simulink subsystem "iLBCReceive"  (R2024b)
settings: Solver=VariableStepAuto  StartTime=0.0  StopTime=10.0  RelTol=1e-3
undefined symbols (not defined in the file or in its folder): ilbc, ilbcMode, Newton, Raphson
libraries: simulink x15, matrix_library x6, dspilbclib x3, dspstat3 x3, dspquant2 x3, dspsigops x2, dspsnks4 x1, simulink_need_slupdate x1, dspobslib x1
settings Model: Creator=fredr  LastModifiedBy=fredr

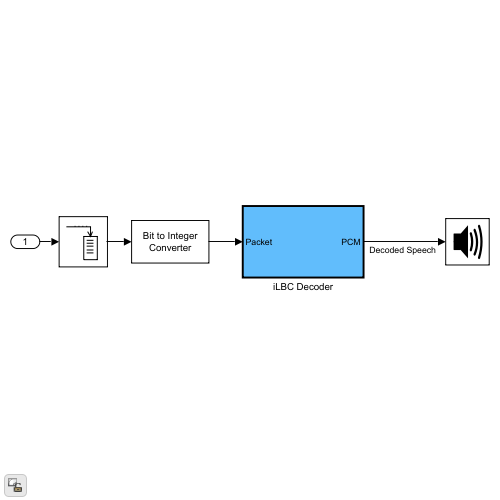
[thumbnail: Simulink's stored preview of the top-level diagram]
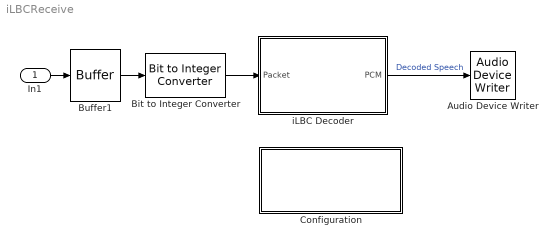
== system iLBCReceive ==
  In1 : Inport
  Audio Device Writer : dspsnks4/Audio Device Writer  Driver=DirectSound  Device=Default  InheritSampleRate=off  SampleRate=8000  BitDepth=16-bit integer  BufferSize=4096  NumBuffers=10  DefaultOutputChannelMapping=on  OutputChannelMapping=1:2  OutputNumUnderrunSamples=off  DriverIdx=1  DeviceWarnFlag=''
  Bit to Integer Converter : simulink/Logic and Bit Operations/Bit to Integer Converter  nbits=8  bitOrder=MSB first  signedOutputValues=Unsigned  outDtype=Inherit via internal rule  outDtypeSigned=Inherit via internal rule
  Buffer1 : Buffer  N=400  OutputFrames=off
  Configuration : Subsystem  mask(iLBC Configuration){ilbcDialogMode=13.33 kbit/sec mode, ilbcDialogDatatype=double}
      mask prompts: ilbcDialogMode "iLBC mode:"; ilbcDialogDatatype "Internal data type:"
      mask help:
      | The iLBC standard is defined for two data rates: 13.33 kbit/sec and 15.20 kbit/sec.  Running under 13.33 kbit/sec, the encoder creates and outputs a compressed speech packet every 30ms.  With the 15.20 kbit/sec data rate, the encoder will output a packet every 20ms.  For the 13.33 kbit/sec mode, the packet size is a uint8 column vector of length 50, where each element represents one byte.  For the 15.20 kbit/sec mode, the packet is of length 38 bytes.
      |
      | The "Internal Data Type" option controls the precision for all internal floating point calculations in the iLBC Encoder and Decoder. The possible options are double and single precision.
      mask init:
      | if ilbcDialogMode == 1
      |     ilbcModeStr = '13.33';
      | elseif ilbcDialogMode == 2
      |     ilbcModeStr = '15.20';
      | end
      | 
      | if ilbcDialogDatatype == 1
      |     ilbcDatatype = 'double';
      | elseif ilbcDialogDatatype == 2
      |     ilbcDatatype = 'single';
      | end
      mask TypeOptions ilbcDialogMode: 13.33 kbit/sec mode | 15.20 kbit/sec mode
      mask TypeOptions ilbcDialogDatatype: double | single
      mask Display:
      | disp([ilbcModeStr ' kb/sec mode\n' ...
      |     'Internal data type: ' ilbcDatatype '\n' ...
      |     '[Double-click to change]']);
  iLBC Decoder : Subsystem  TreatAsAtomicUnit=on
  wires:
  Buffer1/1 -> Bit to Integer Converter/1
  iLBC Decoder/1(PCM) -> Audio Device Writer/1  "Decoded Speech"
  Bit to Integer Converter/1 -> iLBC Decoder/1(Packet)
  In1/1 -> Buffer1/1

== system iLBCReceive/Configuration ==

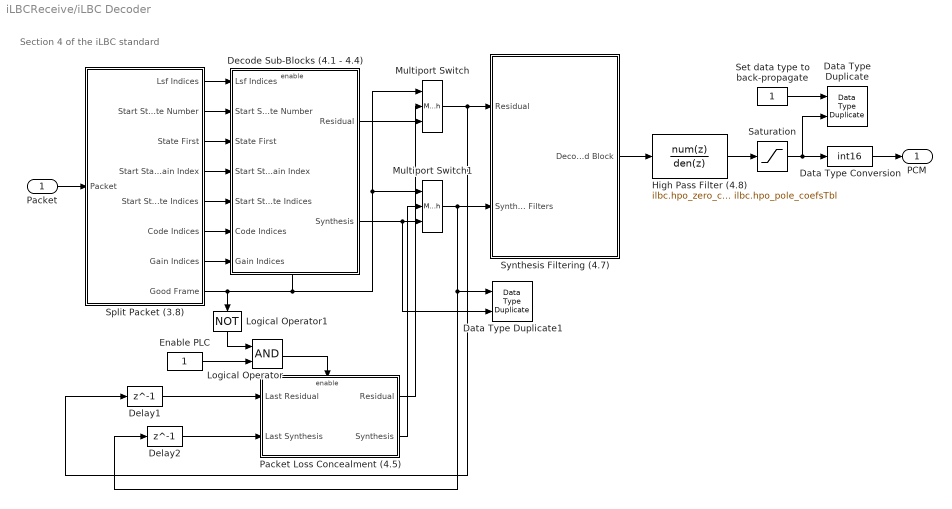
== system iLBCReceive/iLBC Decoder ==
  note: Section 4 of the iLBC standard
  Packet : Inport
  Data Type Duplicate : DataTypeDuplicate
  Data Type Duplicate1 : DataTypeDuplicate
  Data Type Conversion : DataTypeConversion  OutDataTypeStr=int16  RndMeth=Floor
  Decode Sub-Blocks (4.1 - 4.4) : Subsystem
  Delay1 : Delay  DelayLength=1  InitialCondition=0
  Delay2 : Delay  DelayLength=1  InitialCondition=0
  Enable PLC : Constant  OutDataTypeStr=boolean
  High Pass Filter (4.8) : DiscreteFilter  Numerator=ilbc.hpo_zero_coefsTbl  Denominator=ilbc.hpo_pole_coefsTbl  InputProcessing=Columns as channels (frame based)  FilterStructure=Direct form II transposed  a0EqualsOne=on  NumAccumDataTypeStr=Inherit: Same as product output  DenAccumDataTypeStr=Inherit: Same as product output
  Logical Operator : Logic  AllPortsSameDT=off  OutDataTypeStr=boolean
  Logical Operator1 : Logic  Operator=NOT  AllPortsSameDT=off  OutDataTypeStr=boolean
  Multiport Switch : MultiPortSwitch  DataPortOrder=Zero-based contiguous  Inputs=2  zeroidx=on  SaturateOnIntegerOverflow=off  InputSameDT=off
  Multiport Switch1 : MultiPortSwitch  DataPortOrder=Zero-based contiguous  Inputs=2  zeroidx=on  SaturateOnIntegerOverflow=off  InputSameDT=off
  Packet Loss Concealment (4.5) : Subsystem
  Saturation : Saturate  UpperLimit=32767  LowerLimit=-32768
  Set data type to back-propagate : Constant  OutDataTypeStr=ilbcDatatype
  Split Packet (3.8) : Subsystem  TreatAsAtomicUnit=on
  Synthesis Filtering (4.7) : Subsystem  TreatAsAtomicUnit=on
  PCM : Outport  VectorParamsAs1DForOutWhenUnconnected=off
  wires:
  Delay2/1 -> Packet Loss Concealment (4.5)/2(Last Synthesis)
  Multiport Switch1/1 -> Synthesis Filtering (4.7)/2(Synthesis Filters), Data Type Duplicate1/1, Delay2/1
  Delay1/1 -> Packet Loss Concealment (4.5)/1(Last Residual)
  Multiport Switch/1 -> Synthesis Filtering (4.7)/1(Residual), Delay1/1
  High Pass Filter (4.8)/1 -> Saturation/1
  Packet/1 -> Split Packet (3.8)/1(Packet)
  Data Type Conversion/1 -> PCM/1
  Saturation/1 -> Data Type Conversion/1, Data Type Duplicate/2
  Synthesis Filtering (4.7)/1(Decoded Block) -> High Pass Filter (4.8)/1
  Split Packet (3.8)/2(Start State Number) -> Decode Sub-Blocks (4.1 - 4.4)/2(Start State Number)
  Split Packet (3.8)/3(State First) -> Decode Sub-Blocks (4.1 - 4.4)/3(State First)
  Split Packet (3.8)/4(Start State Gain Index) -> Decode Sub-Blocks (4.1 - 4.4)/4(Start State Gain Index)
  Split Packet (3.8)/5(Start State Indices) -> Decode Sub-Blocks (4.1 - 4.4)/5(Start State Indices)
  Split Packet (3.8)/6(Code Indices) -> Decode Sub-Blocks (4.1 - 4.4)/6(Code Indices)
  Split Packet (3.8)/7(Gain Indices) -> Decode Sub-Blocks (4.1 - 4.4)/7(Gain Indices)
  Split Packet (3.8)/1(Lsf Indices) -> Decode Sub-Blocks (4.1 - 4.4)/1(Lsf Indices)
  Split Packet (3.8)/8(Good Frame) -> Logical Operator1/1, Multiport Switch/1, Multiport Switch1/1, Decode Sub-Blocks (4.1 - 4.4)/Enable
  Decode Sub-Blocks (4.1 - 4.4)/1(Residual) -> Multiport Switch/3
  Decode Sub-Blocks (4.1 - 4.4)/2(Synthesis) -> Multiport Switch1/3, Data Type Duplicate1/2
  Packet Loss Concealment (4.5)/1(Residual) -> Multiport Switch/2
  Packet Loss Concealment (4.5)/2(Synthesis) -> Multiport Switch1/2
  Logical Operator/1 -> Packet Loss Concealment (4.5)/Enable
  Logical Operator1/1 -> Logical Operator/1
  Set data type to back-propagate/1 -> Data Type Duplicate/1
  Enable PLC/1 -> Logical Operator/2

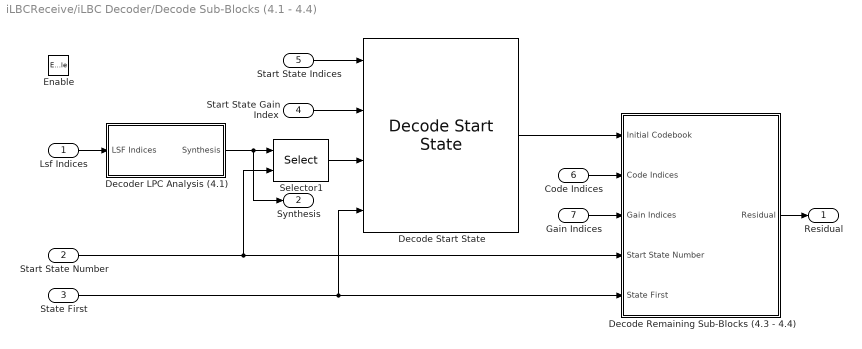
== system iLBCReceive/iLBC Decoder/Decode Sub-Blocks (4.1 - 4.4) ==
  Lsf Indices : Inport
  Start State Number : Inport  Port=2
  State First : Inport  Port=3
  Start State Gain Index : Inport  Port=4
  Start State Indices : Inport  Port=5
  Code Indices : Inport  Port=6
  Gain Indices : Inport  Port=7
  Enable : EnablePort
  Decode Remaining Sub-Blocks (4.3 - 4.4) : Subsystem  TreatAsAtomicUnit=on
  Decode Start State : dspilbclib/Decode Start State  SystemSampleTime=-1  VariantActivationTime=update diagram  AllowFlexibleInterface=on  Latency=0  AutoFrameSizeCalculation=off
  Decoder LPC Analysis (4.1) : Subsystem  TreatAsAtomicUnit=on
  Selector1 : Selector  NumberOfDimensions=2  InputPortWidth=3  IndexOptions=Select all,Index vector (port)  Indices=-1,-1  OutputSizes=1
  Residual : Outport  VectorParamsAs1DForOutWhenUnconnected=off
  Synthesis : Outport  Port=2  VectorParamsAs1DForOutWhenUnconnected=off
  wires:
  Decode Remaining Sub-Blocks (4.3 - 4.4)/1(Residual) -> Residual/1
  Gain Indices/1 -> Decode Remaining Sub-Blocks (4.3 - 4.4)/3(Gain Indices)
  Code Indices/1 -> Decode Remaining Sub-Blocks (4.3 - 4.4)/2(Code Indices)
  Start State Gain Index/1 -> Decode Start State/2
  Start State Indices/1 -> Decode Start State/1
  Decoder LPC Analysis (4.1)/1(Synthesis) -> Selector1/1, Synthesis/1
  Lsf Indices/1 -> Decoder LPC Analysis (4.1)/1(LSF Indices)
  State First/1 -> Decode Remaining Sub-Blocks (4.3 - 4.4)/5(State First), Decode Start State/4
  Selector1/1 -> Decode Start State/3
  Start State Number/1 -> Decode Remaining Sub-Blocks (4.3 - 4.4)/4(Start State Number), Selector1/2
  Decode Start State/1 -> Decode Remaining Sub-Blocks (4.3 - 4.4)/1(Initial Codebook)

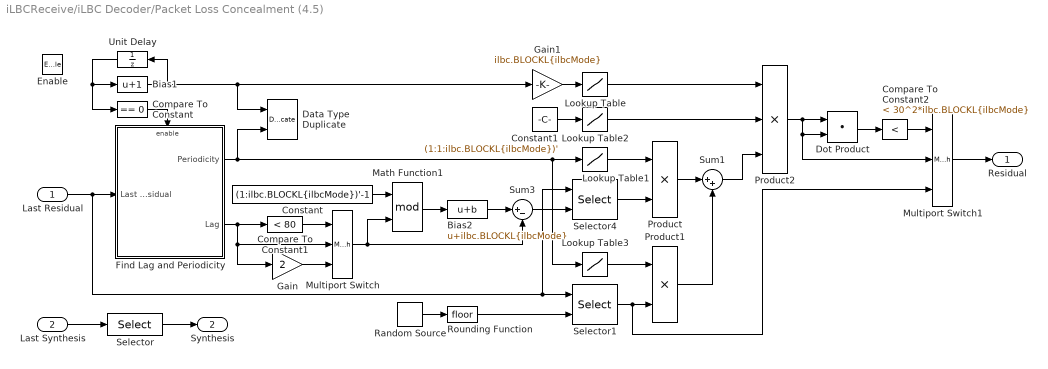
== system iLBCReceive/iLBC Decoder/Packet Loss Concealment (4.5) ==
  Last Residual : Inport
  Last Synthesis : Inport  Port=2
  Enable : EnablePort  StatesWhenEnabling=reset
  Bias1 : Bias  Bias=1  SaturateOnIntegerOverflow=off
  Bias2 : Bias  Bias=ilbc.BLOCKL{ilbcMode}  SaturateOnIntegerOverflow=off
  Compare To Constant : simulink/Logic and Bit Operations/Compare To Constant  relop===  const=0  OutDataTypeStr=boolean  ZeroCross=off
  Compare To Constant1 : simulink/Logic and Bit Operations/Compare To Constant  relop=<  const=80  OutDataTypeStr=uint8  ZeroCross=off
  Compare To Constant2 : simulink/Logic and Bit Operations/Compare To Constant  relop=<  const=30^2*ilbc.BLOCKL{ilbcMode}  OutDataTypeStr=boolean  ZeroCross=off
  Constant : Constant  Value=(1:ilbc.BLOCKL{ilbcMode})'-1  VectorParams1D=off  OutDataTypeStr=Inherit: Inherit via back propagation
  Constant1 : Constant  Value=(1:1:ilbc.BLOCKL{ilbcMode})'  VectorParams1D=off  OutDataTypeStr=Inherit: Inherit via back propagation
  Data Type Duplicate : DataTypeDuplicate
  Dot Product : DotProduct  OutDataTypeStr=Inherit: Inherit via internal rule
  Find Lag and Periodicity : Subsystem  TreatAsAtomicUnit=on
  Gain : Gain  Gain=2  OutDataTypeStr=Inherit: Same as input
  Gain1 : Gain  Gain=ilbc.BLOCKL{ilbcMode}  OutDataTypeStr=Inherit: Inherit via back propagation  ParamDataTypeStr=Inherit: Same as input
  Lookup Table : Lookup_n-D  NumberOfTableDimensions=1  BreakpointsForDimension1=[0 320 640 960 1280]  Table=[1.0 0.9 0.7 0.5 0.0]  InterpMethod=Flat
  Lookup Table1 : Lookup_n-D  NumberOfTableDimensions=1  BreakpointsForDimension1=[0.3 0.6]  Table=[0 1]  ExtrapMethod=Clip
  Lookup Table2 : Lookup_n-D  NumberOfTableDimensions=1  BreakpointsForDimension1=[80 160 240]  Table=[1.00 0.95 0.90]  ExtrapMethod=Clip
  Lookup Table3 : Lookup_n-D  NumberOfTableDimensions=1  BreakpointsForDimension1=[0.3 0.6]  Table=[1 0]  ExtrapMethod=Clip
  Math Function1 : Math  Operator=mod  SignedPower=on
  Multiport Switch : MultiPortSwitch  DataPortOrder=Zero-based contiguous  Inputs=2  zeroidx=on  SaturateOnIntegerOverflow=off  InputSameDT=off
  Multiport Switch1 : MultiPortSwitch  DataPortOrder=Zero-based contiguous  Inputs=2  zeroidx=on  SaturateOnIntegerOverflow=off  InputSameDT=off
  Product : Product  RndMeth=Zero
  Product1 : Product  RndMeth=Zero
  Product2 : Product  Inputs=3  RndMeth=Zero  OutDataTypeStr=Inherit: Same as first input
  Random Source : dspobslib/Random Source  SrcType=Uniform  NormMethod=Ziggurat  CltLength=12  MinVal=ilbc.BLOCKL{ilbcMode}-70  MaxVal=ilbc.BLOCKL{ilbcMode}-0.001  MeanVal=0  VarVal=1  RepMode=Not repeatable  rawSeed=1  IsInherit=off  SampMode=Discrete  SampTime=-1  SampFrame=ilbc.BLOCKL{ilbcMode}  DataType=Single  OutComplex=Real  OutputFrames=off
  Rounding Function : Rounding
  Selector : Selector  NumberOfDimensions=2  InputPortWidth=3  IndexOptions=Select all,Index vector (dialog)  Indices=[1 3],repmat(ilbc.NSUB{ilbcMode},1,ilbc.NSUB{ilbcMode})  OutputSizes=1,1
  Selector1 : Selector  NumberOfDimensions=2  IndexMode=Zero-based  InputPortWidth=3  IndexOptions=Index vector (port),Select all  Indices=[1 3],1  OutputSizes=1,1
  Selector4 : Selector  NumberOfDimensions=2  IndexMode=Zero-based  InputPortWidth=3  IndexOptions=Index vector (port),Select all  Indices=[1 3],1  OutputSizes=1,1
  Sum1 : Sum  Inputs=|++
  Sum3 : Sum  Inputs=|+-
  Unit Delay : UnitDelay  SampleTime=-1  HasFrameUpgradeWarning=on
  Residual : Outport  VectorParamsAs1DForOutWhenUnconnected=off
  Synthesis : Outport  Port=2  VectorParamsAs1DForOutWhenUnconnected=off
  wires:
  Last Synthesis/1 -> Selector/1
  Selector/1 -> Synthesis/1
  Find Lag and Periodicity/2(Lag) -> Compare To Constant1/1, Multiport Switch/2, Gain/1
  Find Lag and Periodicity/1(Periodicity) -> Lookup Table1/1, Lookup Table3/1, Data Type Duplicate/2
  Compare To Constant1/1 -> Multiport Switch/1
  Gain1/1 -> Lookup Table/1
  Constant1/1 -> Lookup Table2/1
  Sum1/1 -> Product2/3
  Dot Product/1 -> Compare To Constant2/1
  Compare To Constant2/1 -> Multiport Switch1/1
  Multiport Switch1/1 -> Residual/1
  Lookup Table/1 -> Product2/1
  Lookup Table2/1 -> Product2/2
  Last Residual/1 -> Find Lag and Periodicity/1(Last Residual), Selector4/1, Selector1/1
  Product2/1 -> Dot Product/1, Dot Product/2, Multiport Switch1/2
  Constant/1 -> Math Function1/1
  Math Function1/1 -> Bias2/1
  Bias2/1 -> Sum3/1
  Sum3/1 -> Selector4/2
  Multiport Switch/1 -> Math Function1/2, Sum3/2
  Lookup Table1/1 -> Product/1
  Selector4/1 -> Product/2
  Lookup Table3/1 -> Product1/1
  Selector1/1 -> Product1/2, Multiport Switch1/3
  Product/1 -> Sum1/1
  Product1/1 -> Sum1/2
  Gain/1 -> Multiport Switch/3
  Random Source/1 -> Rounding Function/1
  Compare To Constant/1 -> Find Lag and Periodicity/Enable
  Unit Delay/1 -> Bias1/1, Compare To Constant/1
  Rounding Function/1 -> Selector1/2
  Bias1/1 -> Unit Delay/1, Gain1/1, Data Type Duplicate/1

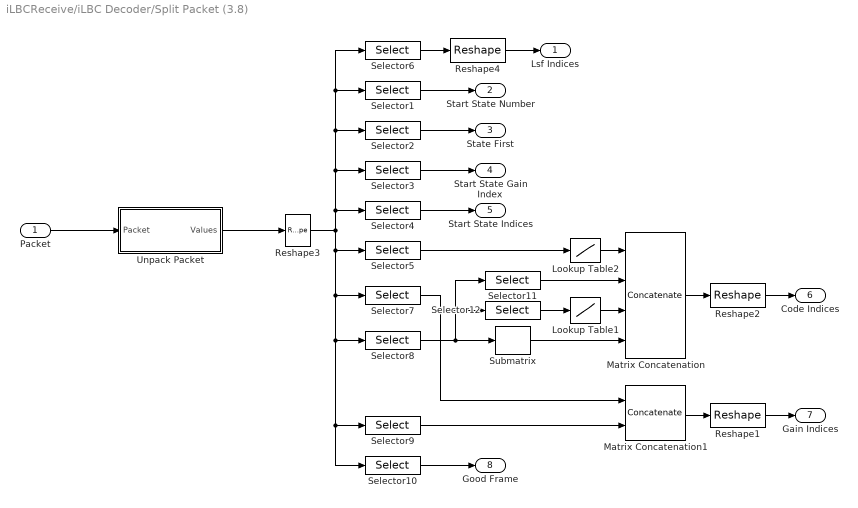
== system iLBCReceive/iLBC Decoder/Split Packet (3.8) ==
  Packet : Inport
  Lookup Table1 : Lookup_n-D  NumberOfTableDimensions=1  BreakpointsForDimension1=[0:255]  Table=[0:43 108:171 236:255 zeros(1,128)]  ExtrapMethod=Clip
  Lookup Table2 : Lookup_n-D  NumberOfTableDimensions=1  BreakpointsForDimension1=[0:255]  Table=[0:57 zeros(1,6) 128:185 zeros(1,134)]  ExtrapMethod=Clip
  Matrix Concatenation : Concatenate  NumInputs=4  Mode=Multidimensional array
  Matrix Concatenation1 : Concatenate  Mode=Multidimensional array
  Reshape1 : Reshape  OutputDimensionality=Customize  OutputDimensions=[3 (ilbc.NSUB{ilbcMode}-1)]
  Reshape2 : Reshape  OutputDimensionality=Customize  OutputDimensions=[3 (ilbc.NSUB{ilbcMode}-1)]
  Reshape3 : Reshape  OutputDimensionality=Column vector (2-D)
  Reshape4 : Reshape  OutputDimensionality=Customize  OutputDimensions=[3 (3-ilbcMode)]
  Selector1 : Selector  NumberOfDimensions=2  InputPortWidth=3  IndexOptions=Index vector (dialog),Select all  Indices=ilbc.packet_idxTbl{ilbcMode}{2},-1  OutputSizes=1
  Selector10 : Selector  NumberOfDimensions=2  InputPortWidth=3  IndexOptions=Index vector (dialog),Select all  Indices=ilbc.packet_idxTbl{ilbcMode}{10},-1  OutputSizes=1
  Selector11 : Selector  NumberOfDimensions=2  InputPortWidth=3  IndexOptions=Index vector (dialog),Select all  Indices=1,-1  OutputSizes=1
  Selector12 : Selector  NumberOfDimensions=2  InputPortWidth=3  IndexOptions=Index vector (dialog),Select all  Indices=2:3,-1  OutputSizes=1
  Selector2 : Selector  NumberOfDimensions=2  InputPortWidth=3  IndexOptions=Index vector (dialog),Select all  Indices=ilbc.packet_idxTbl{ilbcMode}{3},-1  OutputSizes=1
  Selector3 : Selector  NumberOfDimensions=2  InputPortWidth=3  IndexOptions=Index vector (dialog),Select all  Indices=ilbc.packet_idxTbl{ilbcMode}{4},-1  OutputSizes=1
  Selector4 : Selector  NumberOfDimensions=2  InputPortWidth=3  IndexOptions=Index vector (dialog),Select all  Indices=ilbc.packet_idxTbl{ilbcMode}{5},-1  OutputSizes=1
  Selector5 : Selector  NumberOfDimensions=2  InputPortWidth=3  IndexOptions=Index vector (dialog),Select all  Indices=ilbc.packet_idxTbl{ilbcMode}{6},-1  OutputSizes=1
  Selector6 : Selector  NumberOfDimensions=2  InputPortWidth=3  IndexOptions=Index vector (dialog),Select all  Indices=ilbc.packet_idxTbl{ilbcMode}{1},-1  OutputSizes=1
  Selector7 : Selector  NumberOfDimensions=2  InputPortWidth=3  IndexOptions=Index vector (dialog),Select all  Indices=ilbc.packet_idxTbl{ilbcMode}{7},-1  OutputSizes=1
  Selector8 : Selector  NumberOfDimensions=2  InputPortWidth=3  IndexOptions=Index vector (dialog),Select all  Indices=ilbc.packet_idxTbl{ilbcMode}{8},-1  OutputSizes=1
  Selector9 : Selector  NumberOfDimensions=2  InputPortWidth=3  IndexOptions=Index vector (dialog),Select all  Indices=ilbc.packet_idxTbl{ilbcMode}{9},-1  OutputSizes=1
  Submatrix : matrix_library/Submatrix  RowSpan=Range of rows  RowStartMode=Index  RowStartIndex=4  RowEndMode=Last  RowEndIndex=1  ColSpan=All columns  ColStartMode=First  ColStartIndex=1  ColEndMode=Last  ColEndIndex=1
  Unpack Packet : Subsystem  TreatAsAtomicUnit=on
  Lsf Indices : Outport  VectorParamsAs1DForOutWhenUnconnected=off
  Start State Number : Outport  Port=2  VectorParamsAs1DForOutWhenUnconnected=off
  State First : Outport  Port=3  VectorParamsAs1DForOutWhenUnconnected=off
  Start State Gain Index : Outport  Port=4  VectorParamsAs1DForOutWhenUnconnected=off
  Start State Indices : Outport  Port=5  VectorParamsAs1DForOutWhenUnconnected=off
  Code Indices : Outport  Port=6  VectorParamsAs1DForOutWhenUnconnected=off
  Gain Indices : Outport  Port=7  VectorParamsAs1DForOutWhenUnconnected=off
  Good Frame : Outport  Port=8  VectorParamsAs1DForOutWhenUnconnected=off
  wires:
  Matrix Concatenation/1 -> Reshape2/1
  Matrix Concatenation1/1 -> Reshape1/1
  Reshape2/1 -> Code Indices/1
  Reshape1/1 -> Gain Indices/1
  Selector1/1 -> Start State Number/1
  Selector3/1 -> Start State Gain Index/1
  Selector4/1 -> Start State Indices/1
  Selector2/1 -> State First/1
  Selector9/1 -> Matrix Concatenation1/2
  Selector7/1 -> Matrix Concatenation1/1
  Selector10/1 -> Good Frame/1
  Selector6/1 -> Reshape4/1
  Reshape3/1 -> Selector8/1, Selector10/1, Selector9/1, Selector7/1, Selector5/1, Selector4/1, Selector3/1, Selector2/1, Selector6/1, Selector1/1
  Reshape4/1 -> Lsf Indices/1
  Selector5/1 -> Lookup Table2/1
  Selector8/1 -> Selector11/1, Selector12/1, Submatrix/1
  Submatrix/1 -> Matrix Concatenation/4
  Selector11/1 -> Matrix Concatenation/2
  Selector12/1 -> Lookup Table1/1
  Lookup Table2/1 -> Matrix Concatenation/1
  Lookup Table1/1 -> Matrix Concatenation/3
  Packet/1 -> Unpack Packet/1(Packet)
  Unpack Packet/1(Values) -> Reshape3/1

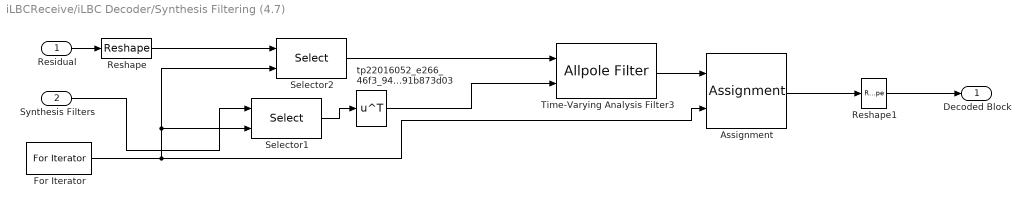
== system iLBCReceive/iLBC Decoder/Synthesis Filtering (4.7) ==
  Residual : Inport
  Synthesis Filters : Inport  Port=2
  Assignment : Assignment  NumberOfDimensions=2  OutputInitialize=Specify size for each dimension in table  IndexOptions=Assign all,Index vector (port)  Indices=-1,1  OutputSizes=40,ilbc.NSUB{ilbcMode}
  For Iterator : ForIterator  IterationLimit=ilbc.NSUB{ilbcMode}  IterationVariableDataType=int8
  Reshape : Reshape  OutputDimensionality=Customize  OutputDimensions=[40 ilbc.NSUB{ilbcMode}]
  Reshape1 : Reshape  OutputDimensionality=Column vector (2-D)  OutputDimensions=[50 4]
  Selector1 : Selector  NumberOfDimensions=2  InputPortWidth=3  IndexOptions=Select all,Index vector (port)  Indices=-1,-1  OutputSizes=1
  Selector2 : Selector  NumberOfDimensions=2  InputPortWidth=3  IndexOptions=Select all,Index vector (port)  Indices=-1,-1  OutputSizes=1
  Time-Varying Analysis Filter3 : AllpoleFilter  CoefSource=Input port  AccumDataTypeStr=Inherit: Same as product output
      settings: InputPortMap=u0,u1
  tp22016052_e266_46f3_948b_11691b873d03 : Math  Operator=transpose  SignedPower=on
  Decoded Block : Outport  VectorParamsAs1DForOutWhenUnconnected=off
  wires:
  tp22016052_e266_46f3_948b_11691b873d03/1 -> Time-Varying Analysis Filter3/2
  Selector1/1 -> tp22016052_e266_46f3_948b_11691b873d03/1
  Residual/1 -> Reshape/1
  Synthesis Filters/1 -> Selector1/1
  Selector2/1 -> Time-Varying Analysis Filter3/1
  For Iterator/1 -> Selector1/2, Selector2/2, Assignment/2
  Reshape/1 -> Selector2/1
  Time-Varying Analysis Filter3/1 -> Assignment/1
  Assignment/1 -> Reshape1/1
  Reshape1/1 -> Decoded Block/1

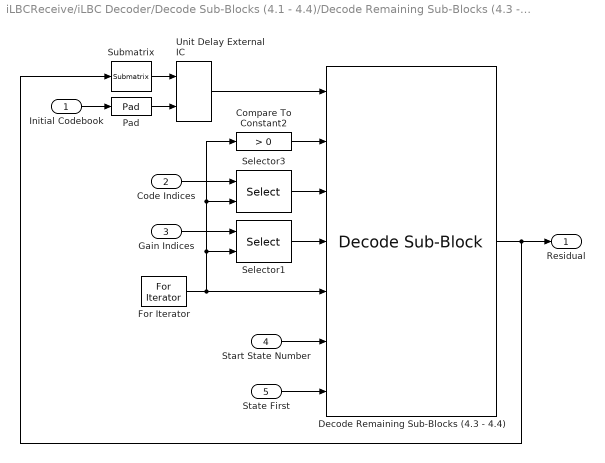
== system iLBCReceive/iLBC Decoder/Decode Sub-Blocks (4.1 - 4.4)/Decode Remaining Sub-Blocks (4.3 - 4.4) ==
  Initial Codebook : Inport
  Code Indices : Inport  Port=2
  Gain Indices : Inport  Port=3
  Start State Number : Inport  Port=4
  State First : Inport  Port=5
  Compare To Constant2 : simulink/Logic and Bit Operations/Compare To Constant  relop=>  const=0  OutDataTypeStr=uint8  ZeroCross=off
  Decode Remaining Sub-Blocks (4.3 - 4.4) : dspilbclib/Decode Sub-Block  SystemSampleTime=-1  VariantActivationTime=update diagram  AllowFlexibleInterface=on  Latency=0  AutoFrameSizeCalculation=off
  For Iterator : ForIterator  ResetStates=reset  IterationLimit=ilbc.NSUB{ilbcMode}-1  IndexMode=Zero-based
  Pad : dspsigops/Pad  padAlong=Columns  dimsToPad=1  valSrc=Specify via dialog  padVal=0  spec=Pad size  padNumOutRowsSpecMethod=User-specified  numOutRows=ilbc.BLOCKL{ilbcMode}-40  padNumOutColsSpecMethod=User-specified  numOutCols=1  isVarDimsMode=off  padBeginning=90  padEnd=0  outSizeMode=User-specified  outSize=1  padSigAt=Beginning  trunc_flag=None  roundingMode=Floor  overflowMode=off  truncOrWrapMode=Truncate  wrap_flag=None
  Selector1 : Selector  NumberOfDimensions=2  IndexMode=Zero-based  InputPortWidth=3  IndexOptions=Select all,Index vector (port)  Indices=-1,0  OutputSizes=1
  Selector3 : Selector  NumberOfDimensions=2  IndexMode=Zero-based  InputPortWidth=3  IndexOptions=Select all,Index vector (port)  Indices=-1,0  OutputSizes=1
  Submatrix : matrix_library/Submatrix  RowSpan=Range of rows  RowStartMode=Index  RowStartIndex=41  RowEndMode=Last  RowEndIndex=1  ColSpan=All columns  ColStartMode=First  ColStartIndex=1  ColEndMode=Last  ColEndIndex=1
  Unit Delay External IC : simulink_need_slupdate/Unit Delay External IC  tsamp=-1
  Residual : Outport  VectorParamsAs1DForOutWhenUnconnected=off
  wires:
  State First/1 -> Decode Remaining Sub-Blocks (4.3 - 4.4)/7
  Start State Number/1 -> Decode Remaining Sub-Blocks (4.3 - 4.4)/6
  Compare To Constant2/1 -> Decode Remaining Sub-Blocks (4.3 - 4.4)/2
  Unit Delay External IC/1 -> Decode Remaining Sub-Blocks (4.3 - 4.4)/1
  Pad/1 -> Unit Delay External IC/2
  Submatrix/1 -> Unit Delay External IC/1
  Initial Codebook/1 -> Pad/1
  Code Indices/1 -> Selector3/1
  Gain Indices/1 -> Selector1/1
  Selector1/1 -> Decode Remaining Sub-Blocks (4.3 - 4.4)/4
  Selector3/1 -> Decode Remaining Sub-Blocks (4.3 - 4.4)/3
  Decode Remaining Sub-Blocks (4.3 - 4.4)/1 -> Residual/1, Submatrix/1
  For Iterator/1 -> Decode Remaining Sub-Blocks (4.3 - 4.4)/5, Selector1/2, Compare To Constant2/1, Selector3/2

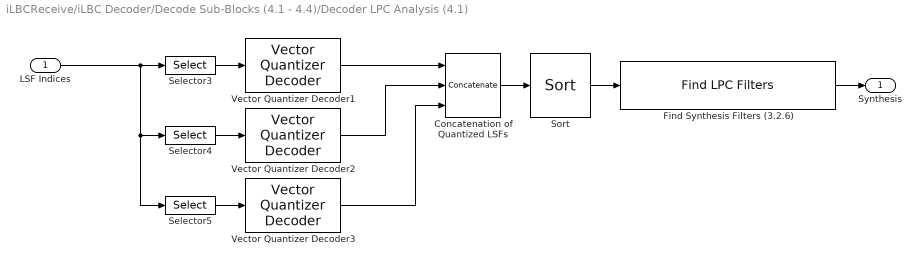
== system iLBCReceive/iLBC Decoder/Decode Sub-Blocks (4.1 - 4.4)/Decoder LPC Analysis (4.1) ==
  LSF Indices : Inport
  Concatenation of Quantized LSFs : Concatenate  NumInputs=3  Mode=Multidimensional array
  Find Synthesis Filters (3.2.6) : dspilbclib/Find LPC Filters  SystemSampleTime=-1  VariantActivationTime=update diagram  AllowFlexibleInterface=on  Latency=0  AutoFrameSizeCalculation=off
  Selector3 : Selector  NumberOfDimensions=2  InputPortWidth=3  IndexOptions=Index vector (dialog),Select all  Indices=1,-1  OutputSizes=1
  Selector4 : Selector  NumberOfDimensions=2  InputPortWidth=3  IndexOptions=Index vector (dialog),Select all  Indices=2,-1  OutputSizes=1
  Selector5 : Selector  NumberOfDimensions=2  InputPortWidth=3  IndexOptions=Index vector (dialog),Select all  Indices=3,-1  OutputSizes=1
  Sort : dspstat3/Sort  otype=Value  dir=Ascending  sortAlg=Quick sort  roundingMode=Floor  overflowMode=off
  Vector Quantizer Decoder1 : dspquant2/Vector Quantizer Decoder  invalidin=Clip  CBsource=Specify via dialog  codebook=ilbc.lsfCbTbl1  dataType=Inherit via back propagation  isSigned=on  wordLen=16  udDataType=float('single')  fracBitsMode=Best precision  numFracBits=7  OutDataTypeStr=Inherit: Inherit via back propagation  LastOutDataTypeStr=Inherit: Inherit via back propagation
  Vector Quantizer Decoder2 : dspquant2/Vector Quantizer Decoder  invalidin=Clip  CBsource=Specify via dialog  codebook=ilbc.lsfCbTbl2  dataType=Inherit via back propagation  isSigned=on  wordLen=16  udDataType=float('single')  fracBitsMode=Best precision  numFracBits=7  OutDataTypeStr=Inherit: Inherit via back propagation  LastOutDataTypeStr=Inherit: Inherit via back propagation
  Vector Quantizer Decoder3 : dspquant2/Vector Quantizer Decoder  invalidin=Clip  CBsource=Specify via dialog  codebook=ilbc.lsfCbTbl3  dataType=Inherit via back propagation  isSigned=on  wordLen=16  udDataType=float('single')  fracBitsMode=Best precision  numFracBits=7  OutDataTypeStr=Inherit: Inherit via back propagation  LastOutDataTypeStr=Inherit: Inherit via back propagation
  Synthesis : Outport  VectorParamsAs1DForOutWhenUnconnected=off
  wires:
  Selector3/1 -> Vector Quantizer Decoder1/1
  Selector4/1 -> Vector Quantizer Decoder2/1
  Selector5/1 -> Vector Quantizer Decoder3/1
  Vector Quantizer Decoder1/1 -> Concatenation of Quantized LSFs/1
  Vector Quantizer Decoder2/1 -> Concatenation of Quantized LSFs/2
  Vector Quantizer Decoder3/1 -> Concatenation of Quantized LSFs/3
  Concatenation of Quantized LSFs/1 -> Sort/1
  Sort/1 -> Find Synthesis Filters (3.2.6)/1
  Find Synthesis Filters (3.2.6)/1 -> Synthesis/1
  LSF Indices/1 -> Selector5/1, Selector4/1, Selector3/1

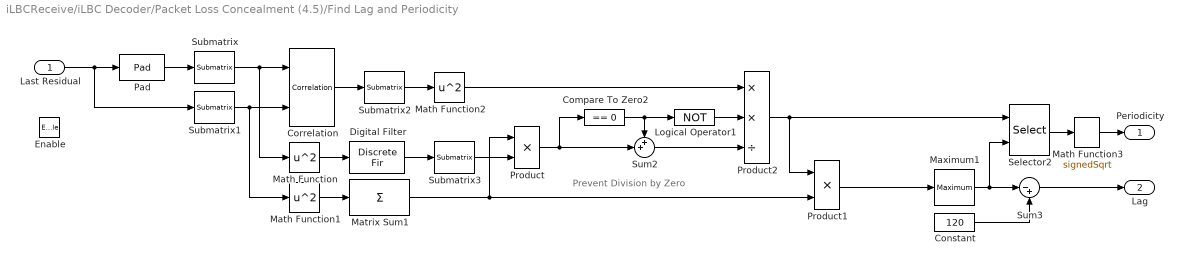
== system iLBCReceive/iLBC Decoder/Packet Loss Concealment (4.5)/Find Lag and Periodicity ==
  note: Prevent Division by Zero
  Last Residual : Inport
  Enable : EnablePort
  Compare To Zero2 : simulink/Logic and Bit Operations/Compare To Zero  relop===  OutDataTypeStr=uint8  ZeroCross=off
  Constant : Constant  Value=120  OutDataTypeStr=Inherit: Inherit via back propagation
  Correlation : dspstat3/Correlation  domain=Time  roundingMode=Floor  overflowMode=off  outputDataTypeStr=Inherit: Same as accumulator  outputMin=[]  outputMax=[]  outputLastDataTypeStr=Inherit: Same as accumulator
  Digital Filter : DiscreteFir  Coefficients=(ones(60,1)).'  InputProcessing=Columns as channels (frame based)  AccumDataTypeStr=Inherit: Same as product output
  Logical Operator1 : Logic  Operator=NOT  AllPortsSameDT=off  OutDataTypeStr=boolean
  Math Function : Math  Operator=square  SignedPower=on
  Math Function1 : Math  Operator=square  SignedPower=on
  Math Function2 : Math  Operator=square  SignedPower=on
  Math Function3 : Sqrt  Operator=signedSqrt  AlgorithmType=Newton-Raphson
  Matrix Sum1 : Sum  Inputs=+  CollapseMode=Specified dimension  OutDataTypeStr=Inherit: Same as accumulator
  Maximum1 : dspstat3/Maximum  operation=maximum  fcn=Index  indexBase=Zero  operateOver=Each column  Dimension=1  InputProcessing=Columns as channels (frame based)  reset=None  roiEnable=off  roiType=Rectangles  roiPortion=Entire ROI  roiOutput=Individual statistics for each ROI  roiFlag=off  roundingMode=Floor  overflowMode=off  accumDataTypeStr=Inherit: Same as product output  accumLastDataTypeStr=Inherit: Same as product output
  Pad : dspsigops/Pad  padAlong=Columns  dimsToPad=1  valSrc=Specify via dialog  padVal=0  spec=Output size  padNumOutRowsSpecMethod=User-specified  numOutRows=60+120  padNumOutColsSpecMethod=User-specified  numOutCols=1  isVarDimsMode=off  padBeginning=0  padEnd=0  outSizeMode=User-specified  outSize=1  padSigAt=Beginning  trunc_flag=None  roundingMode=Floor  overflowMode=off  truncOrWrapMode=Truncate  wrap_flag=None
  Product : Product  RndMeth=Zero
  Product1 : Product  RndMeth=Zero
  Product2 : Product  Inputs=**/  RndMeth=Zero
  Selector2 : Selector  NumberOfDimensions=2  IndexMode=Zero-based  InputPortWidth=3  IndexOptions=Index vector (port),Index vector (dialog)  Indices=[1 3],0  OutputSizes=7,1
  Submatrix : matrix_library/Submatrix  RowSpan=Range of rows  RowStartMode=First  RowStartIndex=120+60-1  RowEndMode=Offset from last  RowEndIndex=20  ColSpan=All columns  ColStartMode=First  ColStartIndex=1  ColEndMode=Last  ColEndIndex=1
  Submatrix1 : matrix_library/Submatrix  RowSpan=Range of rows  RowStartMode=Offset from last  RowStartIndex=60-1  RowEndMode=Last  RowEndIndex=60  ColSpan=All columns  ColStartMode=First  ColStartIndex=1  ColEndMode=Last  ColEndIndex=1
  Submatrix2 : matrix_library/Submatrix  RowSpan=Range of rows  RowStartMode=Index  RowStartIndex=60  RowEndMode=Offset from last  RowEndIndex=60-1  ColSpan=All columns  ColStartMode=First  ColStartIndex=1  ColEndMode=Last  ColEndIndex=1
  Submatrix3 : matrix_library/Submatrix  RowSpan=Range of rows  RowStartMode=Offset from last  RowStartIndex=100  RowEndMode=Last  RowEndIndex=101  ColSpan=All columns  ColStartMode=First  ColStartIndex=1  ColEndMode=Last  ColEndIndex=1
  Sum2 : Sum  Inputs=++|
  Sum3 : Sum  Inputs=|-+
  Periodicity : Outport  VectorParamsAs1DForOutWhenUnconnected=off
  Lag : Outport  Port=2  VectorParamsAs1DForOutWhenUnconnected=off
  wires:
  Last Residual/1 -> Pad/1, Submatrix1/1
  Correlation/1 -> Submatrix2/1
  Submatrix2/1 -> Math Function2/1
  Pad/1 -> Submatrix/1
  Math Function1/1 -> Matrix Sum1/1
  Math Function/1 -> Digital Filter/1
  Digital Filter/1 -> Submatrix3/1
  Matrix Sum1/1 -> Product1/2, Product/1
  Product/1 -> Sum2/2, Compare To Zero2/1
  Sum2/1 -> Product2/3
  Product2/1 -> Product1/1, Selector2/1
  Selector2/1 -> Math Function3/1
  Sum3/1 -> Lag/1
  Submatrix1/1 -> Correlation/2, Math Function1/1
  Submatrix/1 -> Math Function/1, Correlation/1
  Maximum1/1 -> Selector2/2, Sum3/1
  Math Function2/1 -> Product2/1
  Product1/1 -> Maximum1/1
  Constant/1 -> Sum3/2
  Math Function3/1 -> Periodicity/1
  Submatrix3/1 -> Product/2
  Logical Operator1/1 -> Product2/2
  Compare To Zero2/1 -> Logical Operator1/1, Sum2/1

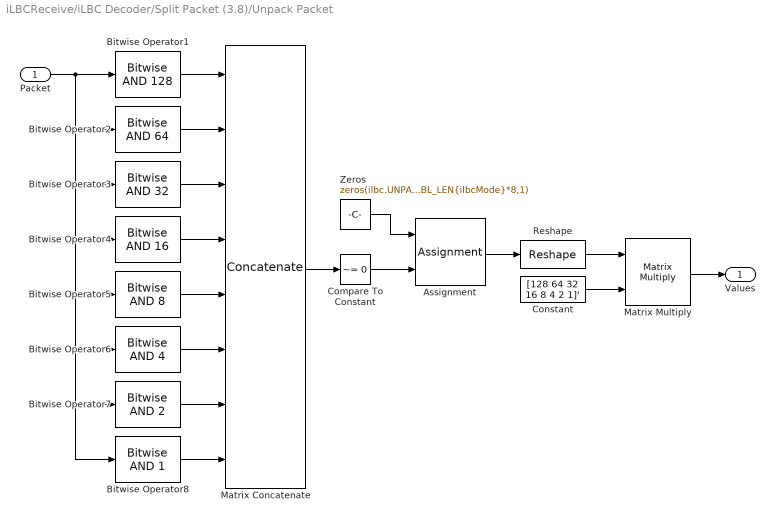
== system iLBCReceive/iLBC Decoder/Split Packet (3.8)/Unpack Packet ==
  Packet : Inport
  Assignment : Assignment  IndexOptions=Index vector (dialog)  Indices=ilbc.bit_packTbl{ilbcMode}  OutputSizes=1
  Bitwise Operator1 : simulink/Logic and Bit Operations/Bitwise Operator  logicop=AND  UseBitMask=on  BitMask=128  BitMaskRealWorld=Stored Integer
  Bitwise Operator2 : simulink/Logic and Bit Operations/Bitwise Operator  logicop=AND  UseBitMask=on  BitMask=64  BitMaskRealWorld=Stored Integer
  Bitwise Operator3 : simulink/Logic and Bit Operations/Bitwise Operator  logicop=AND  UseBitMask=on  BitMask=32  BitMaskRealWorld=Stored Integer
  Bitwise Operator4 : simulink/Logic and Bit Operations/Bitwise Operator  logicop=AND  UseBitMask=on  BitMask=16  BitMaskRealWorld=Stored Integer
  Bitwise Operator5 : simulink/Logic and Bit Operations/Bitwise Operator  logicop=AND  UseBitMask=on  BitMask=8  BitMaskRealWorld=Stored Integer
  Bitwise Operator6 : simulink/Logic and Bit Operations/Bitwise Operator  logicop=AND  UseBitMask=on  BitMask=4  BitMaskRealWorld=Stored Integer
  Bitwise Operator7 : simulink/Logic and Bit Operations/Bitwise Operator  logicop=AND  UseBitMask=on  BitMask=2  BitMaskRealWorld=Stored Integer
  Bitwise Operator8 : simulink/Logic and Bit Operations/Bitwise Operator  logicop=AND  UseBitMask=on  BitMask=1  BitMaskRealWorld=Stored Integer
  Compare To Constant : simulink/Logic and Bit Operations/Compare To Constant  relop=~=  const=0  OutDataTypeStr=boolean  ZeroCross=off
  Constant : Constant  Value=[128 64 32 16 8 4 2 1]'  VectorParams1D=off  OutDataTypeStr=uint8
  Matrix Concatenate : Concatenate  NumInputs=8  Mode=Multidimensional array
  Matrix Multiply : Product  Multiplication=Matrix(*)  OutDataTypeStr=uint8
  Reshape : Reshape  OutputDimensionality=Customize  OutputDimensions=[ilbc.UNPACKED_TBL_LEN{ilbcMode} 8]
  Zeros : Constant  Value=zeros(ilbc.UNPACKED_TBL_LEN{ilbcMode}*8,1)  VectorParams1D=off  OutDataTypeStr=boolean
  Values : Outport  VectorParamsAs1DForOutWhenUnconnected=off
  wires:
  Zeros/1 -> Assignment/1
  Compare To Constant/1 -> Assignment/2
  Assignment/1 -> Reshape/1
  Reshape/1 -> Matrix Multiply/1
  Constant/1 -> Matrix Multiply/2
  Matrix Concatenate/1 -> Compare To Constant/1
  Matrix Multiply/1 -> Values/1
  Packet/1 -> Bitwise Operator1/1, Bitwise Operator2/1, Bitwise Operator8/1, Bitwise Operator7/1, Bitwise Operator6/1, Bitwise Operator5/1, Bitwise Operator4/1, Bitwise Operator3/1
  Bitwise Operator1/1 -> Matrix Concatenate/1
  Bitwise Operator2/1 -> Matrix Concatenate/2
  Bitwise Operator3/1 -> Matrix Concatenate/3
  Bitwise Operator4/1 -> Matrix Concatenate/4
  Bitwise Operator5/1 -> Matrix Concatenate/5
  Bitwise Operator6/1 -> Matrix Concatenate/6
  Bitwise Operator7/1 -> Matrix Concatenate/7
  Bitwise Operator8/1 -> Matrix Concatenate/8
